simulink model "main_lowpath"  (R2026a)
settings: Solver=VariableStepAuto  StopTime=15  FixedStep=params.MPC.dt  RelTol=1e-2
values from neighbouring files (symbols this model uses):
  P_initial = params.Pd_initial + params.Pcm_initial    [setup_lowpath.m]
undefined symbols (not defined in the file or in its folder): params, Ref
(part 1 of 2)
settings Model: Creator=katsu  LastModifiedBy=hoshino

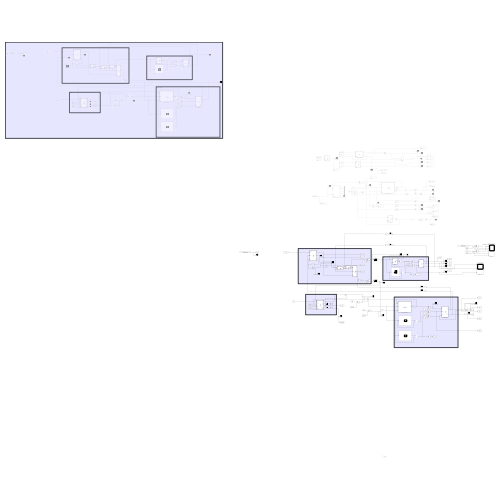
[thumbnail: Simulink's stored preview of the top-level diagram]
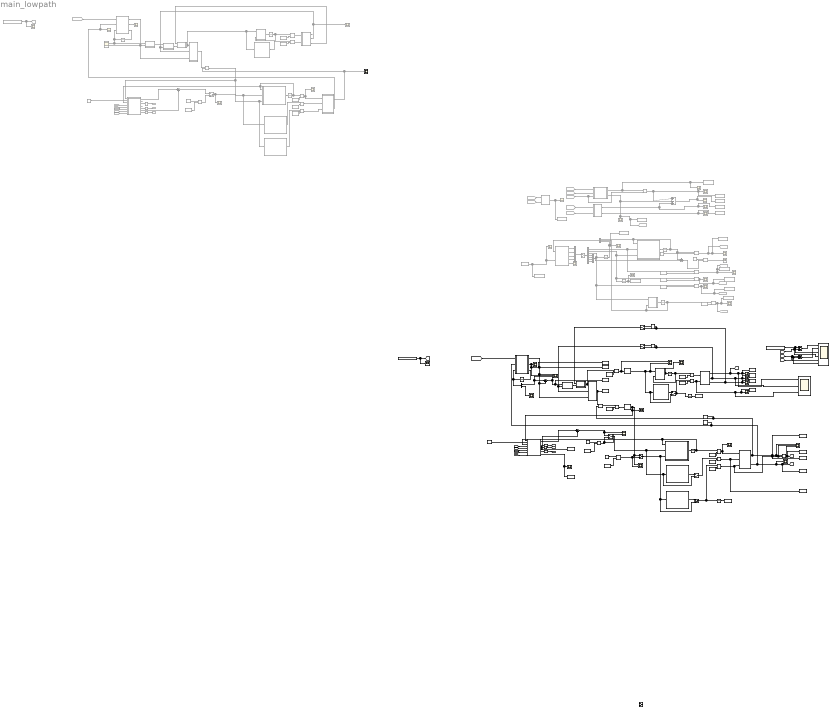
== system main_lowpath ==
  note: Subsystem
  note: NMPC
  note: Power Management
  note: Air Supply System
  note: battery
  note: Air Supply System
  note: NMPC
  note: Power Management
  note: battery
  Add : Sum
  Add1 : Sum
  Air_supply_state : Scope  Commented=on
      settings: ActiveDisplayYMinimum=-1325.34843  ActiveDisplayYMaximum=13777.55778  DataLoggingVariableName=ScopeData3
  Air_supply_state1 : Scope
      settings: ActiveDisplayYMinimum=-8195.03817105226  ActiveDisplayYMaximum=118761.37874277288
  Air_supply_state2 : Scope  Commented=on
      settings: ActiveDisplayYMinimum=-10228.536535853444  ActiveDisplayYMaximum=141574.22093012271  DataLoggingVariableName=ScopeData12
  Air_supply_system : MATLAB Function  Commented=on  TreatAsAtomicUnit=on
  Air_supply_system1 : MATLAB Function  TreatAsAtomicUnit=on
  Air_supply_system2 : MATLAB Function  Commented=on  TreatAsAtomicUnit=on
  Battery : MATLAB Function  Commented=on  TreatAsAtomicUnit=on
  Battery1 : MATLAB Function  TreatAsAtomicUnit=on
  Battery2 : MATLAB Function  Commented=on  TreatAsAtomicUnit=on
  Battery_state : Scope  Commented=on
      settings: ActiveDisplayYMinimum=-0.0625  ActiveDisplayYMaximum=0.5625  DataLoggingVariableName=ScopeData2
  Battery_state1 : Scope  Commented=on
      settings: ActiveDisplayYMinimum=-0.0625  ActiveDisplayYMaximum=0.5625
  Constant : Constant  Commented=on  Value=Ref.x
  Constant1 : Constant  Commented=on  Value=Ref.x
  Constant10 : Constant  Value=Ref.x
  Constant11 : Constant  Value=Ref.Vcm
  Constant12 : Constant  Value=Ref.Ifc
  Constant13 : Constant  Value=Ref.Ib
  Constant14 : Constant  Value=2
  Constant15 : Constant  Commented=on  Value=Ref.x
  Constant16 : Constant  Commented=on  Value=Ref.Vcm
  Constant17 : Constant  Commented=on  Value=Ref.Ifc
  Constant18 : Constant  Commented=on  Value=Ref.Ib
  Constant19 : Constant  Commented=on  Value=2
  Constant2 : Constant  Commented=on  Value=Ref.Vcm
  Constant20 : Constant  Commented=on  Value=100
  Constant21 : Constant  Commented=on  Value=Ref.Vcm
  Constant22 : Constant  Commented=on  Value=params.Smax
  Constant23 : Constant  Commented=on  Value=Ref.Batt
  Constant24 : Constant  Value=Ref.Ifc
  Constant25 : Constant  Value=100
  Constant26 : Constant  Value=Ref.Ifc
  Constant27 : Constant  Value=Ref.Ib
  Constant3 : Constant  Commented=on  Value=Ref.Ifc
  Constant4 : Constant  Value=100
  Constant5 : Constant  Commented=on  Value=Ref.Batt
  Constant6 : Constant  Commented=on  Value=Ref.Ib
  Constant7 : Constant  Value=Ref.Vcm
  Constant8 : Constant  Value=params.Smax
  Constant9 : Constant  Value=Ref.Batt
  Demux : Demux  Outputs=2
  Demux1 : Demux  Commented=on  Outputs=7
  From : From  Commented=on  GotoTag=supply_state
  From Workspace : FromWorkspace  Commented=on  VariableName=Data.demand
  From Workspace1 : FromWorkspace  VariableName=Demandseries
  From Workspace2 : FromWorkspace  Commented=on  VariableName=Demandseries
  From Workspace3 : FromWorkspace  VariableName=Data.demand
  From1 : From  Commented=on  GotoTag=Vcm
  From13 : From  Commented=on  GotoTag=rammda
  From14 : From  Commented=on  GotoTag=Pd
  From15 : From  Commented=on  GotoTag=Pd
  From16 : From  Commented=on  GotoTag=u_bar
  From2 : From  Commented=on  GotoTag=Ifc
  From3 : From  Commented=on  GotoTag=battery_state
  From4 : From  Commented=on  GotoTag=Ib
  From5 : From  Commented=on  GotoTag=supply_state
  From6 : From  Commented=on  GotoTag=Ifc
  From8 : From  Commented=on  GotoTag=u_b
  Goto : Goto  Commented=on  GotoTag=supply_state
  Goto1 : Goto  Commented=on  GotoTag=Vcm
  Goto10 : Goto  Commented=on  GotoTag=u_bar
  Goto11 : Goto  Commented=on  GotoTag=u_b
  Goto12 : Goto  Commented=on  GotoTag=rammda
  Goto13 : Goto  Commented=on  GotoTag=Pd
  Goto2 : Goto  Commented=on  GotoTag=Ifc
  Goto3 : Goto  Commented=on  GotoTag=Ib
  Goto4 : Goto  Commented=on  GotoTag=battery_state
  Goto5 : Goto  Commented=on  GotoTag=Pcm  TagVisibility=global
  IP_ILQR_controller_test : Subsystem  Commented=on
  Ib : Scope  Commented=on
      settings: ActiveDisplayYMinimum=-12.91203  ActiveDisplayYMaximum=41.45646  DataLoggingVariableName=ScopeData3
  Ifc : Scope  Commented=on
      settings: ActiveDisplayYMinimum=31.92108  ActiveDisplayYMaximum=418.48985  DataLoggingVariableName=ScopeData2
  Integrator1 : Integrator  Commented=on  InitialCondition=params.start.Bat./Ref.Batt
  Integrator10 : Integrator  Commented=on  InitialCondition=[P_initial;0]
  Integrator11 : Integrator
  Integrator12 : Integrator
  Integrator2 : Integrator  Commented=on
  Integrator3 : Integrator  Commented=on
  Integrator4 : Integrator  Commented=on  InitialCondition=params.start.x ./[Ref.x]
  Integrator5 : Integrator  InitialCondition=params.start.Bat./Ref.Batt
  Integrator6 : Integrator  InitialCondition=params.start.x ./[Ref.x]
  Integrator7 : Integrator  InitialCondition=[P_initial;0]
  Integrator8 : Integrator  Commented=on  InitialCondition=params.start.Bat./Ref.Batt
  Integrator9 : Integrator  Commented=on  InitialCondition=params.start.x ./[Ref.x]
  LowPath Filter : MATLAB Function  TreatAsAtomicUnit=on
  LowPath Filter1 : MATLAB Function  Commented=on  TreatAsAtomicUnit=on
  MATLAB Function : MATLAB Function  Commented=on  TreatAsAtomicUnit=on
  MATLAB Function1 : MATLAB Function  TreatAsAtomicUnit=on
  MATLAB Function10 : MATLAB Function  Commented=on  TreatAsAtomicUnit=on
  MATLAB Function11 : MATLAB Function  Commented=on  TreatAsAtomicUnit=on
  MATLAB Function2 : MATLAB Function  TreatAsAtomicUnit=on
  MATLAB Function3 : MATLAB Function  TreatAsAtomicUnit=on
  MATLAB Function5 : MATLAB Function  TreatAsAtomicUnit=on
  MATLAB Function6 : MATLAB Function  Commented=on  TreatAsAtomicUnit=on
  MATLAB Function7 : MATLAB Function  Commented=on  TreatAsAtomicUnit=on
  MATLAB Function8 : MATLAB Function  Commented=on  TreatAsAtomicUnit=on
  MATLAB Function9 : MATLAB Function  Commented=on  TreatAsAtomicUnit=on
  Manual Switch : ManualSwitch  Commented=on
  Manual Switch1 : ManualSwitch
  Manual Switch{3..5,8..9,13} (6 alike) : ManualSwitch  CurrentSetting=0
  Manual Switch2 : ManualSwitch  Commented=on  CurrentSetting=0
  Manual Switch6 : ManualSwitch
  Memory1 : Memory  Commented=on  InitialCondition=zeros(params.nc,params.MPC.N+1)  InheritSampleTime=on  LinearizeAsDelay=on
  Memory10 : Memory  InitialCondition=zeros(params.nc,params.MPC.N+1)  InheritSampleTime=on  LinearizeAsDelay=on
  Memory{3,8,11,13..14,16} (6 alike) : Memory
  Memory12 : Memory  Commented=on  InitialCondition=repmat(params.start.Vcm ,1,params.MPC.N)./Ref.Vcm  InheritSampleTime=on  LinearizeAsDelay=on
  Memory15 : Memory  InitialCondition=100
  Memory17 : Memory  InitialCondition=0/Ref.Ib
  Memory18 : Memory  InitialCondition=params.start.Ifc/Ref.Ifc
  Memory2 : Memory  Commented=on
  Memory4 : Memory  InitialCondition=repmat(params.start.Vcm ,1,params.MPC.N)./Ref.Vcm  InheritSampleTime=on  LinearizeAsDelay=on
  Memory5 : Memory  Commented=on
  Memory6 : Memory  Commented=on  InitialCondition=repmat(params.start.Vcm ,1,params.MPC.N)./Ref.Vcm  InheritSampleTime=on  LinearizeAsDelay=on
  Memory7 : Memory  Commented=on
  Memory9 : Memory  InitialCondition=repmat(params.start.Vcm ,1,params.MPC.N)./Ref.Vcm  InheritSampleTime=on  LinearizeAsDelay=on
  Mux : Mux  Commented=on  Inputs=3
  Mux2 : Mux  Commented=on
  Mux3 : Mux  Commented=on
  NMPC : MATLAB Function  TreatAsAtomicUnit=on  SystemSampleTime=params.MPC.dt
  NMPC1 : MATLAB Function  Commented=on  TreatAsAtomicUnit=on  SystemSampleTime=params.MPC.dt
  Pb : Scope  Commented=on
      settings: ActiveDisplayYMinimum=0.3224  ActiveDisplayYMaximum=5.94025  DataLoggingVariableName=ScopeData6
  Pcm : Scope  Commented=on
      settings: ActiveDisplayYMinimum=-1  ActiveDisplayYMaximum=1  DataLoggingVariableName=ScopeData4
  Pfc : Scope  Commented=on
      settings: ActiveDisplayYMinimum=22359.56986  ActiveDisplayYMaximum=56065.27766  DataLoggingVariableName=ScopeData5
  Product{,1..6,13,15,18..20} (12 alike) : Product  Commented=on
  Product{7..11,24} (6 alike) : Product
  Product{12,14,21..23} (5 alike) : Product  Inputs=*/
  Product16 : Product  Commented=on  Inputs=*/
  Product17 : Product  Commented=on  Inputs=*/
  Scope{,1..3,11..13,15..16} (9 alike) : Scope  Commented=on
      Scope settings: ActiveDisplayYMinimum=-1  ActiveDisplayYMaximum=1  DataLoggingVariableName=ScopeData3
      Scope1 settings: ActiveDisplayYMinimum=-0.37216  ActiveDisplayYMaximum=2.27993
      Scope11 settings: ActiveDisplayYMinimum=3016.1171316949331  ActiveDisplayYMaximum=3016.2378115956235  DataLoggingVariableName=ScopeData19
      Scope12 settings: ActiveDisplayYMinimum=0.23333333333333331  ActiveDisplayYMaximum=0.43333333333333335  DataLoggingVariableName=ScopeData20
      Scope13 settings: ActiveDisplayYMinimum=13419.767122907306  ActiveDisplayYMaximum=33419.7671229073  DataLoggingVariableName=ScopeData23
      Scope15 settings: ActiveDisplayYMinimum=-133.74765078370569  ActiveDisplayYMaximum=1241.7624817944677  DataLoggingVariableName=ScopeData25
      Scope16 settings: ActiveDisplayYMinimum=-1  ActiveDisplayYMaximum=1  DataLoggingVariableName=ScopeData26
      Scope2 settings: ActiveDisplayYMinimum=20919.76712  ActiveDisplayYMaximum=45919.76712
      Scope3 settings: ActiveDisplayYMinimum=-0.23032  ActiveDisplayYMaximum=2.07287
  Scope10 : Scope  Commented=on  NumInputPorts=2
      settings: ActiveDisplayYMinimum=-3304.5007884370825  ActiveDisplayYMaximum=29740.4921615073  DataLoggingVariableName=ScopeData18
  Scope{4..7,9,14,17..20,22..23} (12 alike) : Scope
      Scope14 settings: ActiveDisplayYMinimum=-3.9268591988222229E+8  ActiveDisplayYMaximum=4.3632171308856495E+7  DataLoggingVariableName=ScopeData24
      Scope17 settings: ActiveDisplayYMinimum=0.49926560710245876  ActiveDisplayYMaximum=0.50009309298023563  DataLoggingVariableName=ScopeData27
      Scope18 settings: ActiveDisplayYMinimum=-10298.708545561778  ActiveDisplayYMaximum=37636.355108944415  DataLoggingVariableName=ScopeData28
      Scope19 settings: ActiveDisplayYMinimum=0.0045698888131218505  ActiveDisplayYMaximum=0.004903489987575207  DataLoggingVariableName=ScopeData37
      Scope20 settings: ActiveDisplayYMinimum=-730.0186998053116  ActiveDisplayYMaximum=192.22429997836792  DataLoggingVariableName=ScopeData30
      Scope22 settings: ActiveDisplayYMinimum=25369.414740674121  ActiveDisplayYMaximum=41484.637646119059  DataLoggingVariableName=ScopeData22
      Scope23 settings: ActiveDisplayYMinimum=-0.14181027268126462  ActiveDisplayYMaximum=0.42645648104948913  DataLoggingVariableName=ScopeData32
      Scope4 settings: ActiveDisplayYMinimum=-28030.649175223873  ActiveDisplayYMaximum=7598.0295810710186  DataLoggingVariableName=ScopeData7
      Scope5 settings: ActiveDisplayYMinimum=-493.12462637750832  ActiveDisplayYMaximum=3888.977197270392  DataLoggingVariableName=ScopeData9
      Scope6 settings: ActiveDisplayYMinimum=11.976831986533281  ActiveDisplayYMaximum=31.976831986533281  DataLoggingVariableName=ScopeData35
      Scope7 settings: ActiveDisplayYMinimum=20919.767122907306  ActiveDisplayYMaximum=45919.7671229073
      Scope9 settings: ActiveDisplayYMinimum=371.94061892849527  ActiveDisplayYMaximum=381.43610612277689  DataLoggingVariableName=ScopeData21
  Scope21 : Scope  NumInputPorts=2
      settings: ActiveDisplayYMinimum=-55.614452248103404  ActiveDisplayYMaximum=127.88585003554753  DataLoggingVariableName=ScopeData31
  Scope24 : Scope  NumInputPorts=2
      settings: ActiveDisplayYMinimum=0.013278075542177636  ActiveDisplayYMaximum=0.32050039689907467  DataLoggingVariableName=ScopeData33
  Scope8 : Scope  NumInputPorts=3
      settings: ActiveDisplayYMinimum=-2655.29717878666  ActiveDisplayYMaximum=10940.839864293284  DataLoggingVariableName=ScopeData10
  Sum : Sum  Commented=on  Inputs=|+-+
  Sum1 : Sum  Inputs=|++
  Sum2 : Sum  Commented=on  Inputs=|++
  Sum3 : Sum  Commented=on  Inputs=+-
  Sum5 : Sum  Inputs=|-+
  To Workspace : ToWorkspace  Commented=on  VariableName=Vfc  SaveFormat=Timeseries  SampleTime=-1
  To Workspace1 : ToWorkspace  Commented=on  VariableName=Pfc  SaveFormat=Timeseries  SampleTime=-1
  To Workspace10 : ToWorkspace  Commented=on  VariableName=Ib  SaveFormat=Timeseries  SampleTime=-1
  To Workspace11 : ToWorkspace  Commented=on  VariableName=Battery_state  SaveFormat=Timeseries  SampleTime=-1
  To Workspace12 : ToWorkspace  Commented=on  VariableName=S  SaveFormat=Timeseries  SampleTime=-1
  To Workspace13 : ToWorkspace  Commented=on  VariableName=Pd_ref  SaveFormat=Timeseries  SampleTime=-1
  To Workspace14 : ToWorkspace  Commented=on  VariableName=H2  SaveFormat=Timeseries  SampleTime=-1
  To Workspace15 : ToWorkspace  VariableName=sannso  SaveFormat=Timeseries  SampleTime=params.MPC.dt/5
  To Workspace16 : ToWorkspace  VariableName=Pb  SaveFormat=Timeseries  SampleTime=params.MPC.dt/5
  To Workspace17 : ToWorkspace  VariableName=Vb  SaveFormat=Timeseries  SampleTime=params.MPC.dt/5
  To Workspace18 : ToWorkspace  VariableName=SOC  SaveFormat=Timeseries  SampleTime=params.MPC.dt/5
  To Workspace19 : ToWorkspace  VariableName=Ib  SaveFormat=Timeseries  SampleTime=params.MPC.dt/5
  To Workspace2 : ToWorkspace  Commented=on  VariableName=Pd  SaveFormat=Timeseries  SampleTime=-1
  To Workspace20 : ToWorkspace  VariableName=Ifc  SaveFormat=Timeseries  SampleTime=params.MPC.dt/5
  To Workspace21 : ToWorkspace  VariableName=Vfc  SaveFormat=Timeseries  SampleTime=params.MPC.dt/5
  To Workspace22 : ToWorkspace  VariableName=Pcm  SaveFormat=Timeseries  SampleTime=params.MPC.dt/5
  To Workspace23 : ToWorkspace  VariableName=Vcm  SaveFormat=Timeseries  SampleTime=params.MPC.dt/5
  To Workspace24 : ToWorkspace  VariableName=Pfc  SaveFormat=Timeseries  SampleTime=params.MPC.dt/5
  To Workspace25 : ToWorkspace  VariableName=LowPath_Pb  SaveFormat=Timeseries  SampleTime=params.MPC.dt/5
  To Workspace26 : ToWorkspace  VariableName=LowPath_Pfc  SaveFormat=Timeseries  SampleTime=params.MPC.dt/5
  To Workspace27 : ToWorkspace  VariableName=LowPath_P  SaveFormat=Timeseries  SampleTime=params.MPC.dt/5
  To Workspace28 : ToWorkspace  VariableName=u_b  SaveFormat=Timeseries  SampleTime=params.MPC.dt/5
  To Workspace29 : ToWorkspace  VariableName=S  SaveFormat=Timeseries  SampleTime=params.MPC.dt/5
  To Workspace3 : ToWorkspace  Commented=on  VariableName=Pb  SaveFormat=Timeseries  SampleTime=-1
  To Workspace30 : ToWorkspace  VariableName=H2  SaveFormat=Timeseries  SampleTime=params.MPC.dt/5
  To Workspace31 : ToWorkspace  VariableName=LowPath_Pd  SaveFormat=Timeseries  SampleTime=params.MPC.dt/5
  To Workspace4 : ToWorkspace  Commented=on  VariableName=Vb  SaveFormat=Timeseries  SampleTime=-1
  To Workspace5 : ToWorkspace  Commented=on  VariableName=Pcm  SaveFormat=Timeseries  SampleTime=-1
  To Workspace6 : ToWorkspace  Commented=on  VariableName=z  SaveFormat=Timeseries  SampleTime=-1
  To Workspace7 : ToWorkspace  Commented=on  VariableName=Air_supply_state  SaveFormat=Timeseries  SampleTime=-1
  To Workspace8 : ToWorkspace  Commented=on  VariableName=Vcm  SaveFormat=Timeseries  SampleTime=-1
  To Workspace9 : ToWorkspace  Commented=on  VariableName=Ifc  SaveFormat=Timeseries  SampleTime=-1
  Vb : Scope  Commented=on
      settings: ActiveDisplayYMinimum=3.69258  ActiveDisplayYMaximum=3.98749
  Vcm : Scope  Commented=on
      settings: ActiveDisplayYMinimum=85.32914  ActiveDisplayYMaximum=214.9536  DataLoggingVariableName=ScopeData2
  Vfc : Scope  Commented=on
      settings: ActiveDisplayYMinimum=227.63486  ActiveDisplayYMaximum=271.61772
  battery_check : Scope  NumInputPorts=3
      settings: ActiveDisplayYMinimum=-1762.2893176189878  ActiveDisplayYMaximum=247.2652591031719  DataLoggingVariableName=ScopeData36
  fuel_cel_systeml : MATLAB Function  Commented=on  TreatAsAtomicUnit=on
  fuel_cel_systeml1 : MATLAB Function  TreatAsAtomicUnit=on
  fuel_cel_systeml2 : MATLAB Function  Commented=on  TreatAsAtomicUnit=on
  oxygen excess ratio : Scope  Commented=on
      settings: ActiveDisplayYMinimum=0.78654  ActiveDisplayYMaximum=2.85955  DataLoggingVariableName=ScopeData4
  power_demand : Scope  NumInputPorts=4
      settings: ActiveDisplayYMinimum=522.0084973875928  ActiveDisplayYMaximum=5050.4280773785822  DataLoggingVariableName=ScopeData29
  power_result : Scope  NumInputPorts=6
      settings: ActiveDisplayYMinimum=-8972.7725583677584  ActiveDisplayYMaximum=72908.238746639181  DataLoggingVariableName=ScopeData34
  total P : Scope  Commented=on
      settings: ActiveDisplayYMinimum=22814.59335  ActiveDisplayYMaximum=43416.58639
  u_Vcm : Scope  NumInputPorts=2
      settings: ActiveDisplayYMinimum=-0.031961874031496994  ActiveDisplayYMaximum=0.38765686628347312  DataLoggingVariableName=ScopeData8
  wires:
  Battery/1(dBatt) -> Integrator1/1
  Integrator1/1 -> Product6/1, Battery/2(Batt), Mux/2  "Battery_state"
  Air_supply_system/1(dx) -> Integrator4/1
  Demux1/1 -> Product3/1, Air_supply_system/2(Vcm)  "Vcm"
  Integrator4/1 -> Air_supply_system/1(x), Mux/1, Product1/1, Sum3/1
  MATLAB Function7/1(z) -> To Workspace6/1, oxygen excess ratio/1
  Demux1/2 -> Integrator3/1, Product4/1, Air_supply_system/3(Ifc)  "Ifc"
  Mux/1 -> IP_ILQR_controller_test/1(x2)
  Demux1/3 -> Product5/1, Battery/1(Ib), Integrator2/1  "Ib"
  Sum/1 -> To Workspace2/1, total P/1  "Pd"
  Product/1 -> Sum/1, To Workspace1/1, Pfc/1  "Pfc"
  MATLAB Function/1(Pb) -> Sum/3, To Workspace3/1, Pb/1  "Pb"
  fuel_cel_systeml/1(Vfc) -> Vfc/1, To Workspace/1, Product/1  "Vfc"
  fuel_cel_systeml/2(Pcm) -> Sum/2, Goto5/1, To Workspace5/1, Pcm/1
  MATLAB Function/2(Vb) -> To Workspace4/1, Vb/1  "Vb"
  Mux3/1 -> Sum3/2
  Product1/1 -> Goto/1, To Workspace7/1, Air_supply_state/1
  Constant/1 -> Product1/2
  Constant1/1 -> Product2/1
  Sum3/1 -> Product2/2
  Product2/1 -> Scope/1
  Product3/1 -> To Workspace8/1, Goto1/1, Vcm/1
  Product5/1 -> To Workspace10/1, Goto3/1, Ib/1
  Constant3/1 -> Product4/2
  Constant2/1 -> Product3/2
  Constant6/1 -> Product5/2
  Product4/1 -> To Workspace9/1, Goto2/1, Ifc/1
  From2/1 -> Product/2, fuel_cel_systeml/3(Ifc)
  From1/1 -> fuel_cel_systeml/2(Vcm)
  From/1 -> fuel_cel_systeml/1(x)
  From4/1 -> MATLAB Function/2(Ib)
  From3/1 -> MATLAB Function/1(Batt)
  From5/1 -> MATLAB Function7/1(x)
  From6/1 -> MATLAB Function7/2(Ifc)
  Constant5/1 -> Product6/2
  IP_ILQR_controller_test/5(Batt1) -> Battery_state1/1
  Integrator2/1 -> To Workspace12/1, Scope1/1, Mux/3
  Product6/1 -> Goto4/1, To Workspace11/1, Battery_state/1
  From Workspace/1 -> Scope2/1, IP_ILQR_controller_test/2(Pd1), To Workspace13/1
  Integrator3/1 -> Scope3/1, To Workspace14/1
  IP_ILQR_controller_test/2(Ifc1) -> Mux2/2  "Ifc"
  IP_ILQR_controller_test/1(Vcm1) -> Mux2/1  "Vcm"
  IP_ILQR_controller_test/3(Ib1) -> Mux2/3  "Ib"
  IP_ILQR_controller_test/4(Air1) -> Mux2/4
  Mux2/1 -> Manual Switch/1
  Demux1/4 -> Mux3/1
  Demux1/5 -> Mux3/2
  Demux1/6 -> Mux3/3
  Demux1/7 -> Mux3/4
  Manual Switch/1 -> Demux1/1
  MATLAB Function1/2(Vb) -> Manual Switch9/2, Memory14/1, battery_check/2, To Workspace17/1, Scope9/1  "Vb"
  Constant9/1 -> Product7/2
  Integrator5/1 -> Product7/1, Battery1/2(Batt)  "Battery_state"
  Product7/1 -> MATLAB Function1/1(Batt)
  Battery1/1(dBatt) -> Scope23/1, Integrator5/1
  Air_supply_system1/1(dx) -> Integrator6/1
  Integrator6/1 -> Air_supply_system1/1(x), NMPC/3(x), Product8/1
  Constant10/1 -> Product8/2
  Manual Switch1/1 -> Manual Switch4/2, Memory11/1, Air_supply_system1/2(Vcm)
  Product10/1 -> To Workspace20/1, Scope8/2, Product24/2, fuel_cel_systeml1/3(Ifc)  "Ifc"
  Product9/1 -> To Workspace23/1, fuel_cel_systeml1/2(Vcm)
  Product8/1 -> Air_supply_state1/1, fuel_cel_systeml1/1(x)
  Constant11/1 -> Product9/2
  Constant12/1 -> Product10/2
  Product11/1 -> battery_check/3, To Workspace19/1, Scope20/1, MATLAB Function1/2(Ib)  "Ib"
  Constant13/1 -> Product11/2
  MATLAB Function2/1(Pfc) -> Product12/1, To Workspace26/1
  Sum5/1 -> To Workspace25/1, MATLAB Function5/1(Pb_bar), power_demand/4  "Pb_bar"
  MATLAB Function5/1(Ib_bar) -> MATLAB Function3/2(Ib_bar)
  [Pd] -> LowPath Filter/1(Pd_str)
  LowPath Filter/2(Pd) -> To Workspace31/1, power_demand/2, Scope7/1
  LowPath Filter/3(de) -> Integrator7/1
  Integrator7/1 -> LowPath Filter/3(e), Demux/1
  Constant14/1 -> NMPC/2(z_ref)
  NMPC/1(du1) -> Sum1/1
  Constant7/1 -> Product14/2
  Constant4/1 -> Product14/1
  MATLAB Function3/1(Ib) -> Product23/1, MATLAB Function2/1(Ib)  "Ib"
  Product21/1 -> Memory18/1  "Ifc_ref"
  Manual Switch13/1 -> Product11/1, Integrator11/1
  From Workspace1/1 -> Scope22/1, [Pd]
  Constant8/1 -> NMPC/6(Smax)
  NMPC/5(ub1) -> Sum1/2
  NMPC/3(u_bar) -> Memory4/1
  Memory4/1 -> [u_bar]
  [u_bar] -> NMPC/4("u_bar ")
  NMPC/4(u_b) -> To Workspace28/1, Memory9/1
  Memory9/1 -> [u_b]
  [u_b] -> NMPC/7("u_b ")
  NMPC/6(rammda) -> Memory10/1
  Memory10/1 -> [rammda]
  [rammda] -> NMPC/8("rammda ")
  Sum1/1 -> Manual Switch1/1, u_Vcm/1
  Product14/1 -> Manual Switch1/2, u_Vcm/2
  [Pd] -> NMPC/5(Pd)
  MATLAB Function6/1(Pb) -> ?  "Pb"
  MATLAB Function8/1(Pfc) -> Product16/1
  Product13/1 -> fuel_cel_systeml2/3(Ifc)
  Battery2/1(dBatt) -> Integrator8/1
  LowPath Filter1/3(de) -> Integrator10/1
  NMPC1/1(du1) -> Sum2/1
  Integrator10/1 -> LowPath Filter1/3(e), MATLAB Function10/1(e), Scope10/1
  From13/1 -> NMPC1/8("rammda ")
  Memory7/1 -> Product15/1
  Integrator8/1 -> Product18/1, Battery2/2(Batt)  "Battery_state"
  NMPC1/6(ub1) -> Sum2/2
  NMPC1/2(K0) -> ?
  Product17/1 -> Manual Switch2/2
  NMPC1/7(rammda) -> Memory1/1
  From14/1 -> NMPC1/5(Pd)
  fuel_cel_systeml2/2(Pcm) -> Scope11/1, LowPath Filter1/2(Pcm)
  Constant19/1 -> NMPC1/2(z_ref)
  Memory2/1 -> Product20/1
  Product20/1 -> fuel_cel_systeml2/2(Vcm)
  fuel_cel_systeml2/1(Vfc) -> Product16/2, Scope14/1  "Vfc"
  From16/1 -> NMPC1/4("u_bar ")
  From8/1 -> NMPC1/7("u_b ")
  Memory6/1 -> Goto10/1
  MATLAB Function6/3(SOC) -> MATLAB Function9/1(SOC)
  LowPath Filter1/1(P) -> MATLAB Function8/3(P), Scope10/2, MATLAB Function10/2(P)
  Constant16/1 -> Product20/2
  Constant15/1 -> Product19/2
  Memory1/1 -> Goto12/1
  Constant18/1 -> Product15/2
  Product15/1 -> MATLAB Function6/2(Ib)
  Constant22/1 -> NMPC1/6(Smax)
  MATLAB Function10/1(Pb_bar) -> MATLAB Function11/1(Pb_bar)
  Product19/1 -> Air_supply_state2/1, fuel_cel_systeml2/1(x)
  Sum2/1 -> Manual Switch2/1
  MATLAB Function11/1(Ib_bar) -> MATLAB Function9/2(Ib_bar)
  Constant17/1 -> Product13/2
  Product16/1 -> Memory5/1, Air_supply_system2/3(Ifc), NMPC1/1(Ifc)
  NMPC1/5(u_b) -> Memory12/1
  Constant23/1 -> Product18/2
  From15/1 -> LowPath Filter1/1(Pd_str)
  Memory12/1 -> Goto11/1
  Manual Switch2/1 -> Scope12/1, Memory2/1, Air_supply_system2/2(Vcm)
  Constant20/1 -> Product17/1
  NMPC1/4(x_) -> ?
  NMPC1/3(u_bar) -> Memory6/1
  From Workspace2/1 -> Scope16/1, Goto13/1
  Product18/1 -> MATLAB Function6/1(Batt)
  Constant21/1 -> Product17/2
  MATLAB Function6/2(Vb) -> MATLAB Function8/2(Vb), MATLAB Function11/2(Vb), Scope15/1  "Vb"
  LowPath Filter1/2(Pd) -> Scope13/1
  MATLAB Function9/1(Ib) -> Memory7/1, Battery2/1(Ib), MATLAB Function8/1(Ib)
  Air_supply_system2/1(dx) -> Integrator9/1
  Integrator9/1 -> Air_supply_system2/1(x), NMPC1/3(x), Product19/1
  Memory5/1 -> Product13/1
  Demux/1 -> power_demand/3, Sum5/1  "e1 [Pfc_bar]"
  Demux/2 -> Scope18/1  "e2 [dPfc_bar]"
  LowPath Filter/1(P) -> power_demand/1, Sum5/2, MATLAB Function2/3(P), To Workspace27/1
  MATLAB Function1/1(Pb) -> [Pb], battery_check/1, To Workspace16/1, Scope4/1  "Pb"
  Memory11/1 -> Manual Switch4/1
  Manual Switch4/1 -> Product9/1
  Memory3/1 -> Manual Switch3/1
  Memory8/1 -> Manual Switch13/1
  MATLAB Function1/3(SOC) -> Manual Switch8/2, Memory13/1, To Workspace18/1, Scope17/1
  Manual Switch8/1 -> MATLAB Function3/1(SOC)
  Manual Switch9/1 -> MATLAB Function2/2(Vb), MATLAB Function5/2(Vb)
  fuel_cel_systeml1/1(Vfc) -> Product12/2, Memory15/1, To Workspace21/1, Scope8/1, Product24/1  "Vfc"
  fuel_cel_systeml1/2(Pcm) -> Scope5/1, To Workspace22/1, [Pcm], Memory16/1, LowPath Filter/2(Pcm)  "Pcm"
  Constant24/1 -> Product21/2
  Product12/1 -> Product21/1  "Ifc"
  Manual Switch6/1 -> Manual Switch3/2, Memory3/1, Air_supply_system1/3(Ifc)
  Product22/1 -> Scope24/2, Manual Switch6/2
  Constant25/1 -> Product22/1
  Constant26/1 -> Product22/2
  Memory14/1 -> Manual Switch9/1
  Memory13/1 -> Manual Switch8/1
  Memory17/1 -> Manual Switch13/2, Memory8/1, Scope21/2, Battery1/1(Ib)  "Ib_ref_memory"
  Memory18/1 -> Manual Switch6/1, Scope24/1, NMPC/1(Ifc), Scope19/1
  Product23/1 -> Scope21/1, Memory17/1  "Ib_ref"
  Constant27/1 -> Product23/2
  Add/1 -> power_result/1  "all_demand"
  From Workspace3/1 -> power_result/3, Add/1  "Pd"
  [Pcm] -> power_result/4, Add/2  "Pcm"
  Product24/1 -> Scope8/3, To Workspace24/1, [Pfc]  "Pfc"
  [Pfc] -> power_result/6, Add1/2  "Pfc"
  Add1/1 -> power_result/2  "all_supply"
  [Pb] -> power_result/5, Add1/1  "Pb"
  NMPC/7(sannso) -> To Workspace15/1, Scope6/1
  Integrator11/1 -> To Workspace29/1
  Manual Switch3/1 -> Integrator12/1, Product10/1
  Integrator12/1 -> To Workspace30/1

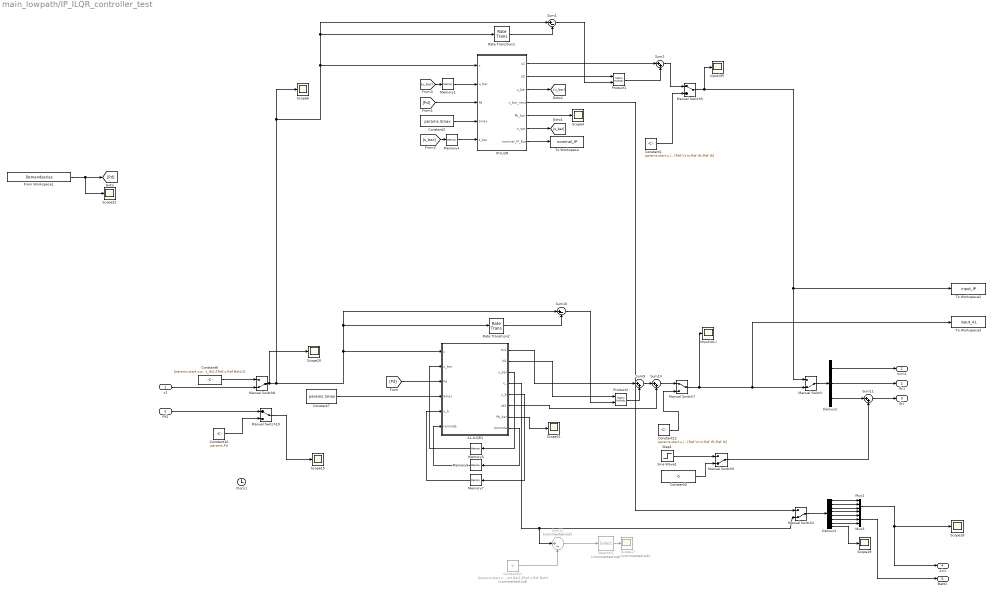
== system main_lowpath/IP_ILQR_controller_test ==
  x2 : Inport
  Pd1 : Inport  Port=2
  AL-ILQR1 : MATLAB Function  TreatAsAtomicUnit=on  SystemSampleTime=params.MPC.dt
  Clock1 : Clock
  Constant1 : Constant  Value=params.start.u./[Ref.Vcm;Ref.Ifc;Ref.Ib]
  Constant10 : Constant  Value=params.Pd
  Constant11 : Constant  Commented=on  Value=[params.start.x;params.start.Bat]./[Ref.x;Ref.Batt]
  Constant12 : Constant  Value=params.start.u./[Ref.Vcm;Ref.Ifc;Ref.Ib]
  Constant2 : Constant  Value=params.Smax
  Constant6 : Constant  Value=[params.start.x;params.start.Bat;params.start.int_Ifc]./[Ref.x;Ref.Batt;1]
  Constant7 : Constant  Value=params.Smax
  Constant9 : Constant  Value=0
  Demux2 : Demux  Outputs=3
  Demux3 : Demux  Outputs=8
  From Workspace1 : FromWorkspace  VariableName=Demandseries
  IP-ILQR : MATLAB Function  TreatAsAtomicUnit=on  SystemSampleTime=params.MPC.dt
  Imput(AL) : Scope
      settings: ActiveDisplayYMinimum=-0.2  ActiveDisplayYMaximum=1.2  DataLoggingVariableName=input_AL
  Input(IP) : Scope
      settings: TimeSpan=5  ActiveDisplayYMinimum=-0.2  ActiveDisplayYMaximum=1.2  DataLoggingVariableName=input_IP
  Manual Switch{,2,8..9} (4 alike) : ManualSwitch  CurrentSetting=0
  Manual Switch10 : ManualSwitch
  Manual Switch3 : ManualSwitch
  Manual Switch7 : ManualSwitch
  Memory1 : Memory  InitialCondition=repmat(params.start.u ,1,params.MPC.N)./[Ref.Vcm;Ref.Ifc;Ref.Ib]  InheritSampleTime=on  LinearizeAsDelay=on
  Memory4 : Memory  InitialCondition=params.start.s  InheritSampleTime=on  LinearizeAsDelay=on
  Memory5 : Memory  InitialCondition=repmat(params.start.u ,1,params.MPC.N)./[Ref.Vcm;Ref.Ifc;Ref.Ib]  InheritSampleTime=on  LinearizeAsDelay=on
  Memory6 : Memory  InitialCondition=zeros(params.nc,params.MPC.N+1)  InheritSampleTime=on  LinearizeAsDelay=on
  Memory7 : Memory  InitialCondition=repmat(params.start.u ,1,params.MPC.N)./[Ref.Vcm;Ref.Ifc;Ref.Ib]  InheritSampleTime=on  LinearizeAsDelay=on
  Mux2 : Mux
  Mux3 : Mux  Inputs=3
  Product1 : Product  Multiplication=Matrix(*)
  Product2 : Product  Multiplication=Matrix(*)
  Rate Transition1 : RateTransition  OutPortSampleTime=params.MPC.dt
  Rate Transition2 : RateTransition  OutPortSampleTime=params.MPC.dt
  Scope{4,6,15,18..22} (8 alike) : Scope
      Scope15 settings: ActiveDisplayYMinimum=-1  ActiveDisplayYMaximum=1  DataLoggingVariableName=ScopeData11
      Scope18 settings: ActiveDisplayYMinimum=-0.12272  ActiveDisplayYMaximum=1.39941  DataLoggingVariableName=ScopeData14
      Scope19 settings: ActiveDisplayYMinimum=-0.01265  ActiveDisplayYMaximum=0.11382  DataLoggingVariableName=ScopeData15
      Scope20 settings: ActiveDisplayYMinimum=-0.15593  ActiveDisplayYMaximum=1.40334  DataLoggingVariableName=ScopeData16
      Scope21 settings: ActiveDisplayYMinimum=-194.73385  ActiveDisplayYMaximum=1761.44655  DataLoggingVariableName=ScopeData17
      Scope22 settings: ActiveDisplayYMinimum=-1  ActiveDisplayYMaximum=1
      Scope4 settings: ActiveDisplayYMinimum=-2111.11617  ActiveDisplayYMaximum=1957.87921  DataLoggingVariableName=ScopeData2
      Scope6 settings: ActiveDisplayYMinimum=-0.37396  ActiveDisplayYMaximum=3.36567
  Scope17 : Scope  Commented=on
      settings: ActiveDisplayYMinimum=-344.77426  ActiveDisplayYMaximum=3043.62299  DataLoggingVariableName=ScopeData13
  Selector1 : Selector  Commented=on  InputPortWidth=7  IndexOptions=Index vector (dialog)  Indices=[1:4 1]  OutputSizes=1
  Sine Wave1 : Sin  Amplitude=10/Ref.Ib  SampleTime=0
  Step1 : Step  Time=3  InitialValue=-10  FinalValue=10  SampleTime=0
  Sum1 : Sum  Inputs=|+-
  Sum10 : Sum  Inputs=|+-
  Sum{2,9,11,13} (4 alike) : Sum  Inputs=|++
  Sum12 : Sum  Commented=on  Inputs=|+-
  To Workspace : ToWorkspace  VariableName=nominal_IP  SaveFormat=Timeseries  SampleTime=-1
  To Workspace2 : ToWorkspace  VariableName=input_IP  SaveFormat=Timeseries  SampleTime=-1
  To Workspace3 : ToWorkspace  VariableName=input_AL  SaveFormat=Timeseries  SampleTime=-1
  Vcm1 : Outport
  Ifc1 : Outport  Port=2
  Ib1 : Outport  Port=3
  Air1 : Outport  Port=4
  Batt1 : Outport  Port=5
  wires:
  Manual Switch3/1 -> To Workspace2/1, Manual Switch/1, Input(IP)/1
  Constant11/1 -> Sum12/2
  AL-ILQR1/6(ub1) -> Sum13/2
  Sum10/1 -> Product2/2
  AL-ILQR1/5(u_b) -> Memory7/1
  AL-ILQR1/3(u_bar) -> Memory5/1
  Sine Wave1/1 -> Manual Switch9/1
  Demux3/2 -> Mux2/2
  Demux3/5 -> Mux3/1
  Memory7/1 -> AL-ILQR1/5("u_b ")
  AL-ILQR1/2(K0) -> Product2/1
  Constant9/1 -> Manual Switch9/2
  Memory6/1 -> AL-ILQR1/6("rammda ")
  Constant7/1 -> AL-ILQR1/4(Smax)
  Sum13/1 -> Manual Switch7/1
  AL-ILQR1/4(x_) -> Manual Switch2/2, Sum12/1
  Constant12/1 -> Manual Switch7/2
  Demux3/8 -> Scope19/1
  AL-ILQR1/8(rammda) -> Memory6/1
  Demux3/3 -> Mux2/3
  Sum11/1 -> Ib1/1
  Sum9/1 -> Sum13/1
  Demux3/4 -> Mux2/4
  Demux2/1 -> Vcm1/1
  Pd1/1 -> Manual Switch10/1
  AL-ILQR1/1(du1) -> Sum9/1
  Memory5/1 -> AL-ILQR1/2("u_bar ")
  Constant6/1 -> Manual Switch8/1
  Demux3/7 -> Mux3/3
  Mux2/1 -> Scope18/1, Air1/1
  Demux2/2 -> Ifc1/1
  Demux3/1 -> Mux2/1
  Demux3/6 -> Mux3/2
  Selector1/1 -> Scope17/1
  Constant10/1 -> Manual Switch10/2
  Product2/1 -> Sum9/2
  Manual Switch7/1 -> To Workspace3/1, Manual Switch/2, Imput(AL)/1
  x2/1 -> Manual Switch8/2
  Manual Switch10/1 -> Scope15/1
  Rate Transition2/1 -> Sum10/2
  Mux3/1 -> Batt1/1
  Demux2/3 -> Sum11/1
  AL-ILQR1/7(Pb_bar) -> Scope21/1
  Sum12/1 -> Selector1/1
  Manual Switch9/1 -> Sum11/2
  Manual Switch/1 -> Demux2/1
  Manual Switch2/1 -> Demux3/1
  IP-ILQR/4(x_bar_next) -> Manual Switch2/1
  Constant1/1 -> Manual Switch3/2
  Sum1/1 -> Product1/2
  IP-ILQR/5(Pb_bar) -> Scope4/1
  Constant2/1 -> IP-ILQR/4(Smax)
  Memory1/1 -> IP-ILQR/2("u_bar ")
  IP-ILQR/2(K0) -> Product1/1
  Sum2/1 -> Manual Switch3/1
  Rate Transition1/1 -> Sum1/2
  Product1/1 -> Sum2/2
  Manual Switch8/1 -> Scope20/1, Scope6/1, Sum1/1, Rate Transition1/1, IP-ILQR/1(x), Sum10/1, Rate Transition2/1, AL-ILQR1/1(x)
  [Pd] -> IP-ILQR/3(Pd)
  [Pd] -> AL-ILQR1/3(Pd)
  From Workspace1/1 -> Scope22/1, [Pd]
  Memory4/1 -> IP-ILQR/5(s_bar)
  IP-ILQR/1(u1) -> Sum2/1
  IP-ILQR/7(nominal_IP_Bus) -> To Workspace/1
  IP-ILQR/6(s_opt) -> [s_bar]
  [s_bar] -> Memory4/1
  IP-ILQR/3(u_bar) -> [u_bar]
  [u_bar] -> Memory1/1

== matlab function main_lowpath/Air_supply_system2 ==
  data: x input; Vcm input; dx output size=4; Ifc input; params parameter; Ref parameter
function dx = Air_supply_4d(x,Vcm,Ifc,params,Ref)
%saturation
% if Vcm < 0  
%    Vcm = 150;
% elseif Vcm > params.Vcm_u/Ref.Vcm 
%    Vcm = params.Vcm_u/Ref.Vcm ;
% end
% 
% if Ifc < 0 
%     Ifc = 0;
% elseif Ifc > 2.2*params.Afc/Ref.Ifc   
%     Ifc = 2.2*params.Afc/Ref.Ifc;
% end

if params.c11/(x(1)+x(2)+params.c2/Ref.pres)>params.c19*Ref.pres
    dx = Air_supply_case1(x,[Vcm;Ifc],[0;0]);
else
    dx = Air_supply_case2(x,[Vcm;Ifc],[0;0]);
end

% x = x./[Ref.x];
% Vcm = Vcm./Ref.Vcm;
% Ifc = Ifc./Ref.Ifc;
% dx = dx.*[Ref.x];

% R_= 8.314;  %Universal gas constant
% patm = 1.01325e5;  %Atomospheric pressure
% psat = 4.736e4;  %Saturation pressure 353K 
% Tatm = 298.15;   %Atmosphric temperature
% Tst = 353.15;    %Temperature of fuel-cell stack 
% Mo2 = 32e-3; %Molar mass of oxygen
% Mn2 = 28e-3; %Molar mass of nitrogen
% Mv = 18.02e-3; %Molar mass of vapour
% Maatm = 28.97e-3; %Molar mass of atmospheric air
% gam = 1.4;  %Air specific heat ratio
% Cp = 1004;   %Air specific ratio
% F = 96487;  %Faraday's constant
% kt = 0.0153;    %motor constant
% kv = 0.0153;    %motor constant
% Rcm = 0.82;    %motor constant
% Jcp = 5e-5;     %compressor and motor interia
% eata_cp = 0.80; %Compressor efficiency
% eata_cm = 0.98; %Compressor motor mechanical efficiency
% n = 381;    %Number of cells in fuel-cell stack
% Afc = 280;   %Fuel-cell active area (cm^2)
% Vsm = 0.02;     %Supply manifold volume
% Vca = 0.01;     %Single stack cathode volume
% kcain = 0.3629e-5; %Cathode inlet orifice
% tm = 1.275e-4;
% Cd = 0.0124;    %Cathode output throttle discharge cofficient
% At = 0.002;     %Cathode output throttle area
% phi_atm = 0.5;  %Average ambient air relative humidity
% yo2atm = 0.21;  %Oxygen molar ratio at cathode inlet
% xo2atm =yo2atm*Mo2/(yo2atm*Mo2+(1-yo2atm)*Mn2); %Oxygen mass fraction at cathode inlet
% watm =Mv/(yo2atm*Mo2+(1-yo2atm)*Mn2)*(phi_atm*psat/(patm-phi_atm*psat)); %Humidity ratio of inlet air
% Kapper = sqrt(mean([Mo2^2,Mn2^2,Mv^2]));
% Vcm_u = 300;
% 
% c1 = (R_*Tst*kcain)/(Mo2*Vca)*(xo2atm/(1+watm));
% c2 = psat;
% c3 = R_*Tst/Vca;
% c4 = Mo2;
% c5 = Mn2;
% c6 = Mv*psat;
% c7 = (R_*Tst*n)/(4*Vca*F);
% c8 = (R_*Tst*kcain)/(Mn2*Vca)*((1-xo2atm)/(1+watm));
% c9 = eata_cm*kt*kv/(Jcp*Rcm);
% c10 = Cp*Tatm/(Jcp*eata_cp);
% c11 = patm;
% c12 = (gam-1/gam);
% c13 = eata_cm*kt/(Jcp*Rcm);
% c14 = R_*Tatm/(Maatm*Vsm);
% c15 = 1/eata_cp;
% c16 = kcain;
% c17 = (Cd*At)/sqrt(R_*Tst)*sqrt(2*gam/(gam-1));
% c18 = 1/gam;
% c19 = (2/(gam+1))^(gam/(gam-1));
% c20 = (Cd*At)/sqrt(R_*Tst)*gam^(1/2)*(2/(gam+1))^((gam+1)/2*(gam-1));
% c21 = 1/Rcm;
% c22 = kv;
% c23 = kcain*xo2atm/(1+watm);
% c24 = n*Mo2/(4*F);
% 
% 
% if c11/(x(1)+x(2)+c2) > c19
% dx = [
%     c1*(-x(1)-x(2)+x(4)-c2)-(c3*x(1)*psi_case1(x,c2,c11,c12,c17,c18,c19,c20))/(c4*x(1)+c5*x(2)+c6)-c7*Ifc;
%     c8*(-x(1)-x(2)+x(4)-c2)-(c3*x(2)*psi_case1(x,c2,c11,c12,c17,c18,c19,c20))/(c4*x(1)+c5*x(2)+c6);
%     -c9*x(3)-(c10./x(3))*((x(4)./c11).^c12-1)*Weight_flow(x(3),x(4))+c13*Vcm;
%     c14*(1+c15*((x(4)./c11)^c12-1))*(Weight_flow(x(3),x(4))-c16*(-x(1)-x(2)+x(4)-c2))];
% else
% 
% dx =  [
%     c1*(-x(1)-x(2)+x(4)-c2)-(c3*x(1)*psi_case2(x,c2,c11,c12,c17,c18,c19,c20))/(c4*x(1)+c5*x(2)+c6)-c7*Ifc;
%     c8*(-x(1)-x(2)+x(4)-c2)-(c3*x(2)*psi_case2(x,c2,c11,c12,c17,c18,c19,c20))/(c4*x(1)+c5*x(2)+c6);
%     -c9*x(3)-(c10./x(3))*((x(4)./c11).^c12-1)*Weight_flow(x(3),x(4))+c13*Vcm;
%     c14*(1+c15*((x(4)./c11)^c12-1))*(Weight_flow(x(3),x(4))-c16*(-x(1)-x(2)+x(4)-c2))];
% end
% 
% 
% 
% 
% %%%%%%%%%%%%%%%%%%%%%%%%%%%%%%%%%%%%%%%%%%%%%%%%%%%%%%%%%%%%%%%%%%%%%%%%%%%%
% 
% end
% 
% function psi = psi_case1(x,c2,c11,c12,c17,c18,c19,c20)
% psi = c17*(x(1)+x(2)+c2)*(c11/(x(1)+x(2)+c2))^c18*sqrt(1-(c11/(x(1)+x(2)+c2))^c12);
% end
% 
% function psi = psi_case2(x,c2,c11,c12,c17,c18,c19,c20)
% psi = c20*(x(1)+x(2)+c2);
% end

== matlab function main_lowpath/Air_supply_system ==
  data: x input; Vcm input; dx output size=4; Ifc input; params parameter; Ref parameter
function dx = Air_supply_4d(x,Vcm,Ifc,params,Ref)
%saturation
% if Vcm < 0  
%    Vcm = 150;
% elseif Vcm > params.Vcm_u/Ref.Vcm 
%    Vcm = params.Vcm_u/Ref.Vcm ;
% end
% 
% if Ifc < 0 
%     Ifc = 0;
% elseif Ifc > 2.2*params.Afc/Ref.Ifc   
%     Ifc = 2.2*params.Afc/Ref.Ifc;
% end

if params.c11/(x(1)+x(2)+params.c2/Ref.pres)>params.c19*Ref.pres
    dx = Air_supply_case1(x,[Vcm;Ifc],[0;0]);
else
    dx = Air_supply_case2(x,[Vcm;Ifc],[0;0]);
end

% x = x./[Ref.x];
% Vcm = Vcm./Ref.Vcm;
% Ifc = Ifc./Ref.Ifc;
% dx = dx.*[Ref.x];

% R_= 8.314;  %Universal gas constant
% patm = 1.01325e5;  %Atomospheric pressure
% psat = 4.736e4;  %Saturation pressure 353K 
% Tatm = 298.15;   %Atmosphric temperature
% Tst = 353.15;    %Temperature of fuel-cell stack 
% Mo2 = 32e-3; %Molar mass of oxygen
% Mn2 = 28e-3; %Molar mass of nitrogen
% Mv = 18.02e-3; %Molar mass of vapour
% Maatm = 28.97e-3; %Molar mass of atmospheric air
% gam = 1.4;  %Air specific heat ratio
% Cp = 1004;   %Air specific ratio
% F = 96487;  %Faraday's constant
% kt = 0.0153;    %motor constant
% kv = 0.0153;    %motor constant
% Rcm = 0.82;    %motor constant
% Jcp = 5e-5;     %compressor and motor interia
% eata_cp = 0.80; %Compressor efficiency
% eata_cm = 0.98; %Compressor motor mechanical efficiency
% n = 381;    %Number of cells in fuel-cell stack
% Afc = 280;   %Fuel-cell active area (cm^2)
% Vsm = 0.02;     %Supply manifold volume
% Vca = 0.01;     %Single stack cathode volume
% kcain = 0.3629e-5; %Cathode inlet orifice
% tm = 1.275e-4;
% Cd = 0.0124;    %Cathode output throttle discharge cofficient
% At = 0.002;     %Cathode output throttle area
% phi_atm = 0.5;  %Average ambient air relative humidity
% yo2atm = 0.21;  %Oxygen molar ratio at cathode inlet
% xo2atm =yo2atm*Mo2/(yo2atm*Mo2+(1-yo2atm)*Mn2); %Oxygen mass fraction at cathode inlet
% watm =Mv/(yo2atm*Mo2+(1-yo2atm)*Mn2)*(phi_atm*psat/(patm-phi_atm*psat)); %Humidity ratio of inlet air
% Kapper = sqrt(mean([Mo2^2,Mn2^2,Mv^2]));
% Vcm_u = 300;
% 
% c1 = (R_*Tst*kcain)/(Mo2*Vca)*(xo2atm/(1+watm));
% c2 = psat;
% c3 = R_*Tst/Vca;
% c4 = Mo2;
% c5 = Mn2;
% c6 = Mv*psat;
% c7 = (R_*Tst*n)/(4*Vca*F);
% c8 = (R_*Tst*kcain)/(Mn2*Vca)*((1-xo2atm)/(1+watm));
% c9 = eata_cm*kt*kv/(Jcp*Rcm);
% c10 = Cp*Tatm/(Jcp*eata_cp);
% c11 = patm;
% c12 = (gam-1/gam);
% c13 = eata_cm*kt/(Jcp*Rcm);
% c14 = R_*Tatm/(Maatm*Vsm);
% c15 = 1/eata_cp;
% c16 = kcain;
% c17 = (Cd*At)/sqrt(R_*Tst)*sqrt(2*gam/(gam-1));
% c18 = 1/gam;
% c19 = (2/(gam+1))^(gam/(gam-1));
% c20 = (Cd*At)/sqrt(R_*Tst)*gam^(1/2)*(2/(gam+1))^((gam+1)/2*(gam-1));
% c21 = 1/Rcm;
% c22 = kv;
% c23 = kcain*xo2atm/(1+watm);
% c24 = n*Mo2/(4*F);
% 
% 
% if c11/(x(1)+x(2)+c2) > c19
% dx = [
%     c1*(-x(1)-x(2)+x(4)-c2)-(c3*x(1)*psi_case1(x,c2,c11,c12,c17,c18,c19,c20))/(c4*x(1)+c5*x(2)+c6)-c7*Ifc;
%     c8*(-x(1)-x(2)+x(4)-c2)-(c3*x(2)*psi_case1(x,c2,c11,c12,c17,c18,c19,c20))/(c4*x(1)+c5*x(2)+c6);
%     -c9*x(3)-(c10./x(3))*((x(4)./c11).^c12-1)*Weight_flow(x(3),x(4))+c13*Vcm;
%     c14*(1+c15*((x(4)./c11)^c12-1))*(Weight_flow(x(3),x(4))-c16*(-x(1)-x(2)+x(4)-c2))];
% else
% 
% dx =  [
%     c1*(-x(1)-x(2)+x(4)-c2)-(c3*x(1)*psi_case2(x,c2,c11,c12,c17,c18,c19,c20))/(c4*x(1)+c5*x(2)+c6)-c7*Ifc;
%     c8*(-x(1)-x(2)+x(4)-c2)-(c3*x(2)*psi_case2(x,c2,c11,c12,c17,c18,c19,c20))/(c4*x(1)+c5*x(2)+c6);
%     -c9*x(3)-(c10./x(3))*((x(4)./c11).^c12-1)*Weight_flow(x(3),x(4))+c13*Vcm;
%     c14*(1+c15*((x(4)./c11)^c12-1))*(Weight_flow(x(3),x(4))-c16*(-x(1)-x(2)+x(4)-c2))];
% end
% 
% 
% 
% 
% %%%%%%%%%%%%%%%%%%%%%%%%%%%%%%%%%%%%%%%%%%%%%%%%%%%%%%%%%%%%%%%%%%%%%%%%%%%%
% 
% end
% 
% function psi = psi_case1(x,c2,c11,c12,c17,c18,c19,c20)
% psi = c17*(x(1)+x(2)+c2)*(c11/(x(1)+x(2)+c2))^c18*sqrt(1-(c11/(x(1)+x(2)+c2))^c12);
% end
% 
% function psi = psi_case2(x,c2,c11,c12,c17,c18,c19,c20)
% psi = c20*(x(1)+x(2)+c2);
% end

== matlab function main_lowpath/Battery ==
  data: Ib input; Batt input; dBatt output; Ref parameter
function dBatt = fcn(Ib,Batt,Ref)
% if Ib <-36/Ref.Ib
%     Ib = -36/Ref.Ib;
% elseif Ib > 36/Ref.Ib
%     Ib = 36/Ref.Ib;
% end
Ib = Ib/15; %pararel 15

dBatt = Battery(Batt,Ib,0);
% Vsoc = Batt(1);
% Vs = Batt(2);
% Vf = Batt(3);

% Cb = 3060;
% SOC = Vsoc*100;
% Rsd = 10e9;
% Rs = 0.3208*exp(-29.14*SOC) +0.04669;
% Cs = -752.9*exp(-13.51*SOC) + 703.6;
% Rf = 6.603*exp(-155.2*SOC) +0.04984;
% Cf = -6056*exp(-27.12*SOC) + 4475;
% 
% 
% dVsoc = -Vsoc/(Rsd*Cb)-Ib/Cb;
% dVs = -Vs/(Rs*Cs)+Ib/Cs;
% dVf = -Vf/(Rf*Cf)+Ib/Cf;
% 
% dBatt = [dVsoc;dVs;dVf];

== matlab function main_lowpath/LowPath Filter ==
  data: P output; Pd output; Pd_str input; de output; Pcm input; e input; params parameter
function [P,Pd,de] = fcn(Pd_str,Pcm,e,params)
% w_n = 2;
% zeta = 1;

w_n = params.w_n;
zeta = params.zeta;
% シミュレーション時間が切り悪いときなにかする必要あり
Pd  = Pd_str(1);
P = Pd + Pcm;
e1 = e(1);
e2 = e(2);

% 論文の式14
% % % % % % % % % % % % % % % % % % % % % % 
de1 = e2;
de2 = -w_n^2*e1 -2*w_n*zeta*e2 + w_n^2*P; % 最後の項はzetaでなくw_n?
% % % % % % % % % % % % % % % % % % % % % % 
de = [de1;de2];
end

== matlab function main_lowpath/IP_ILQR_controller_test/AL-ILQR1 ==
  data: x input size=params.nx; u_bar input size=[params.nu,params.MPC.N]; du1 output size=params.nu; Pd input; K0 output size=[params.nu,params.nx]; u_bar output size=[params.nu,params.MPC.N]; params parameter; x_ output size=params.nx; Ref parameter; Smax input; u_b input; u_b output; ub1 output size=[params.nu 1]; Pb_bar output size=1; rammda input; rammda output
function [du1,K0,u_bar,x_,u_b,ub1,Pb_bar,rammda] = ILQR(x,u_bar,Pd,params,Ref,Smax,u_b,rammda)
% function [du1,K0,u_bar,x_,u_b,ub1,Pb_bar,rammda, nominal_AL_Bus] = ILQR(x,u_bar,Pd,params,Ref,Smax,u_b,rammda)
%UNTITLED3 この関数の概要をここに記述
%   詳細説明をここに記述
du = u_bar-u_b;
% which discretization method
D_method = 'V';                 % D:difference, V:variational


%%%%%%%%%%%%%%%%%%%%%% MPC setting %%%%%%%%%%%%%%%%%%%%%%%%%%%%%%%%%%%%%%%%
% linesearch off:0 on:1
linesearch = 1;
tsp = params.MPC.dt;            % sampling period
N = 10;                         % number of horizon 
N_iter = params.N_iter;         % number of N_iter


nx = size(x,1);                 
nu = size(u_b,1);             
K0 = zeros(nu,nx);             
x_bar = zeros(nx,N+1);
x_opt = zeros(nx,N+1);
%%%%%%%%%%%%%%%%% Augumented Lagrangian setting %%%%%%%%%%%%%%%%%%%%%%%%%%%
nc = 15 ;
nc_i = params.nc_i;
Altro.mu = repmat(4e-4,nc,N+1);
Altro.I_mu = zeros(nc,(N+1)*nc);
Altro.rammda = rammda;
Altro.rammda = zeros(nc,N+1);
Altro.cmax = 1e-8;
Altro.phi = 2;
Value_c = ones(nc,N+1);

for i = 1:N_iter

     for ii = 1:N+1
         for jj = 1:nc
                if Value_c(jj,ii) < 0 && Altro.rammda(jj,ii) == 0 && jj <= nc_i
                    Altro.I_mu(jj,nc*(ii-1)+jj) = 0;
                else
                    Altro.I_mu(jj,nc*(ii-1)+jj) = Altro.mu(jj,ii);
                if Altro.mu(jj,ii)<=100
                    Altro.mu(jj,ii) = Altro.mu(jj,ii)*Altro.phi;
                end
                end

         end
    end

          %disp('AL--------------')
          %disp(i)


    [x_bar,A,B] = forwardpass(x,u_b,du,tsp,N,D_method,params,Ref);
    [du,K0] = backwardpass_Altro_e(x_bar,u_b,du,A,B,N,tsp,linesearch,Pd,params,Altro,Ref,Smax,u_b);
    % [x_bar,A,B] = forwardpass_runge(x,u_b,du,tsp,N,D_method,params,Ref);
    % [du,x_opt, K0] = backwardpass_Altro_e_runge(x_bar,u_b,du,A,B,N,tsp,linesearch,Pd,params,Altro,Ref,Smax);
        for ii = 1:N+1

            if ii ~= N+1
                [x_bar(:,ii),du(:,ii)] = satulation(x_bar(:,ii),u_b(:,ii),du(:,ii));
                if (x_bar(1,:)/0.1173+params.psat/Ref.pres) < 2
                    Value_c(:,ii) = constraints_case1(x_bar(:,ii),u_b(:,ii),du(:,ii),Pd(ii),Smax);
                else
                    Value_c(:,ii) = constraints_case2(x_bar(:,ii),u_b(:,ii),du(:,ii),Pd(ii),Smax);
                end
            else
                [x_bar(:,ii),~] = satulation(x_bar(:,ii),u_b(:,ii-1),du(:,ii-1));
                if (x_bar(1,:)/0.1173+params.psat/Ref.pres) < 2
                    Value_c(:,ii) = constraints_case1(x_bar(:,ii),u_b(:,ii-1),du(:,ii-1),Pd(ii-1),Smax);
                else
                    Value_c(:,ii) = constraints_case2(x_bar(:,ii),u_b(:,ii-1),du(:,ii-1),Pd(ii-1),Smax);
                end
            end

            for jj = 1:nc

                if Value_c(jj,ii) < 0 && Altro.rammda(jj,ii) == 0 && jj <= nc_i
                    Altro.rammda(jj,ii) = max([Altro.rammda(jj,ii) + Altro.mu(jj,ii).*Value_c(jj,ii),0]);
                elseif jj>nc_i
                    Altro.rammda(jj,ii) = Altro.rammda(jj,ii) + Altro.mu(jj,ii).*Value_c(jj,ii);
                else
                end

            end
            % disp(Altro.rammda(:,ii))
        end
end
rammda = circshift(Altro.rammda,-1,2);
rammda(:,end) = rammda(:,end-1);

    % % % % % % % % % % % % % % % % % % % % % % % 
    % % rungeのとき以外に使うとエラーが出る
    % nominal_AL_Bus.u_b = u_b;
    % nominal_AL_Bus.du = du;
    % nominal_AL_Bus.K0 = K0;
    % nominal_AL_Bus.x_opt = x_opt; 
    % nominal_AL_Bus.rammda = rammda;
    % % % % % % % % % % % % % % % % % % % % % % % 



% 制御入力
x_ = x_bar(:,2);
Pb_bar = Pb_fun(x_bar(:,1),u_b(:,1),du(:,1));
du1 = du(:,1);
ub1 = u_b(:,1);

% ノミナルな入力の更新
u_b = u_b+du;
u_bar = circshift(u_b,-1,2);
u_bar(:,end) = u_b(:,end-1);

== matlab function main_lowpath/MATLAB Function7 ==
  data: x input; Ifc input; z output; params parameter
function z = fcn(x,Ifc,params)

z = params.c23*(x(4)-x(1)-x(2)-params.c2)/(params.c24*Ifc);

== matlab function main_lowpath/Battery1 ==
  data: Ib input; Batt input; dBatt output; Ref parameter; params parameter
function dBatt = fcn(Ib,Batt,Ref,params)
% if Ib <-36/Ref.Ib
%     Ib = -36/Ref.Ib;
% elseif Ib > 36/Ref.Ib
%     Ib = 36/Ref.Ib;
% end

n_parallel = params.battery.parallel;
% Ib = Ib/15; %parallel 15
% Battery() already converts pack current to cell current. 

dBatt = Battery(Batt,Ib,0);
% Vsoc = Batt(1);
% Vs = Batt(2);
% Vf = Batt(3);

% Cb = 3060;
% SOC = Vsoc*100;
% Rsd = 10e9;
% Rs = 0.3208*exp(-29.14*SOC) +0.04669;
% Cs = -752.9*exp(-13.51*SOC) + 703.6;
% Rf = 6.603*exp(-155.2*SOC) +0.04984;
% Cf = -6056*exp(-27.12*SOC) + 4475;
% 
% 
% dVsoc = -Vsoc/(Rsd*Cb)-Ib/Cb;
% dVs = -Vs/(Rs*Cs)+Ib/Cs;
% dVf = -Vf/(Rf*Cf)+Ib/Cf;
% 
% dBatt = [dVsoc;dVs;dVf];

== matlab function main_lowpath/MATLAB Function1 ==
  data: Batt input; Pb output; Ib input; Vb output; SOC output; params parameter
function [Pb,Vb,SOC] = fcn(Batt,Ib,params)

n_parallel = params.battery.parallel;
n_series = params.battery.series;
% Ib = Ib/15; %parallel
Ib = Ib/n_parallel;

Vsoc = Batt(1);
Vs = Batt(2);
Vf = Batt(3);
SOC = Vsoc ;
Voc = -1.031*exp(-35*SOC)+3.685+0.2156*SOC-0.1178*SOC^2+0.3201*SOC^3;
R0 = 0.1562*exp(-24.37*SOC)+0.07446;
Vb = Voc-R0*Ib-Vs-Vf;

%Vb = 4;

% セルからパッケージの量へ変換
% Vb = Vb*12;
% Ib = Ib*15;
% Pb = Ib*Vb; %series 12

Vb = Vb*n_series;
Ib = Ib*n_parallel;
Pb = Ib*Vb; %series 12

== matlab function main_lowpath/MATLAB Function5 ==
  data: Pb_bar input; Ib_bar output; Vb input
function Ib_bar = fcn(Pb_bar,Vb)

% 単純な割り算だと数値的に不安定になる test2
%Vb = max(Vb, 0.1);
Ib_bar = Pb_bar/Vb;


% 二次式からIbを計算する．test1
% Vpseudo = Vb;
% R0 = 0.05; %とりあえずこの値にしてみる
% D = Vpseudo^2 - 4 * R0 * Pb_bar;
% 
%     if D < 0
%         % 解なし（物理的にその電力は出せない限界を超えている）
%         % 限界値を出力するか、エラー処理をする
%         Ib_bar = Vpseudo / (2 * R0); % とりあえず頂点の電流値を返す
%     else
%         % 二次方程式の解の公式
%         % 通常、電圧が高い（電流が小さい）方の解が物理的に正しい
%         Ib_bar = (Vpseudo - sqrt(D)) / (2 * R0);
%     end

end

== matlab function main_lowpath/MATLAB Function2 ==
  data: Ib input; Pfc output; Vb input; P input
function Pfc = fcn(Ib,Vb,P)

Pb = Ib*Vb;
Pfc = P - Pb; % P = Pd + Pcm
end

== matlab function main_lowpath/MATLAB Function3 ==
  data: SOC input; Ib_bar input; Ib output
function Ib = fcn(SOC, Ib_bar)
% SOCによってはIb_barに調整を入れる
Ib = Ib_bar;
end
